simulink model "project2_trial_quiz"  (R2018b)
settings: Solver=VariableStepAuto  StartTime=0.0  StopTime=100  RelTol=1e-3
libraries: simulink x1
settings Model: Creator=Ismael  LastModifiedBy=Ismael

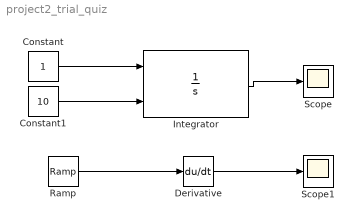
== system project2_trial_quiz ==
  Constant : Constant
  Constant1 : Constant  Value=10
  Derivative : Derivative
  Integrator : Integrator  InitialConditionSource=external
  Ramp : simulink/Sources/Ramp  slope=1  start=0  InitialOutput=0
  Scope : Scope
  Scope1 : Scope
  wires:
  Constant/1 -> Integrator/1
  Integrator/1 -> Scope/1
  Derivative/1 -> Scope1/1
  Ramp/1 -> Derivative/1
  Constant1/1 -> Integrator/2
